simulink model "PI_Controller_sim"  (R2021a)
settings: Solver=ode23t  StartTime=0.0  StopTime=Tsim  RelTol=1e-3  EnableMultiTasking=on
values from neighbouring files (symbols this model uses):
  fo = 50    [PI_Controller.m]    (also in RL_Controller_train.m)
  Iref = 2*Pref/Vg    [PI_Controller.m]    (also in RL_Controller_train.m)
  Ka = -0.05866    [PI_Controller.m]
  Kb = 0.049031    [PI_Controller.m]
  L = 15e-3    (= 0.015)    [PI_Controller.m]    (also in RL_Controller_train.m)
  R = 1e-3    (= 0.001)    [PI_Controller.m]    (also in RL_Controller_train.m)
  Tc = 1/fpwm    (= 5e-05)    [PI_Controller.m]    (also in RL_Controller_train.m)
  Ts = 1/fs    (= 2.5e-05)    [PI_Controller.m]    (also in RL_Controller_train.m)
  Tstep = Ts/500    (= 5e-08)    [RL_Controller_train.m]
  Vdc = 400    [PI_Controller.m]    (also in RL_Controller_train.m)
  Vg = 240*sqrt(2)    [PI_Controller.m]    (also in RL_Controller_train.m)
libraries: spsIGBTDiodeLib x4, spsVoltageMeasurementLib x2, simulink x1, spsDCVoltageSourceLib x1, spsSeriesRLCBranchLib x1, spsACVoltageSourceLib x1, spsGroundLib x1, spsCurrentMeasurementLib x1, spspowerguiLib x1
settings Model: Creator=Ricardo  LastModifiedBy=ASUS-PC
settings SolverCC: AlgebraicLoopSolver=TrustRegion
settings DataIOCC: LimitDataPoints=on  SaveFormat=Array  ReturnWorkspaceOutputs=off
settings OptimizationCC: LifeSpan=inf
settings DebuggingCC: SolverPrmCheckMsg=warning  SFUnexpectedBacktrackingDiag=warning  SFNoUnconditionalDefaultTransitionDiag=warning  SFExecutionAtInitializationDiag=none  SFMachineParentedDataDiag=warning  ArithmeticOperatorsInVariantConditions=warning
settings HardwareCC: ProdBitPerPointer=32  ProdBitPerSizeT=32  ProdBitPerPtrDiffT=32  ProdLargestAtomicFloat=None  ProdIntDivRoundTo=Undefined  ProdEndianess=Unspecified  ProdWordSize=32  ProdHWDeviceType=32-bit Generic
settings ModelReferenceCC: PropagateSignalLabelsOutOfModel=off
settings SFSimCC: SimUseLocalCustomCode=off  CustomCodeUndefinedFunction=UseInterfaceOnly
settings RTWCC: RTWUseLocalCustomCode=off
settings CodeAppCC: StateflowObjectComments=on
settings GRTTargetCC: TargetLangStandard=C89/C90 (ANSI)
settings ConfigComp: CovMetricSettings=dw  CovSaveCumulativeToWorkspaceVar=on  CovSaveSingleToWorkspaceVar=on  CovExternalEMLEnable=off  CovSFcnEnable=off
settings SimscapeCC: SimscapeNormalizeSystem=off

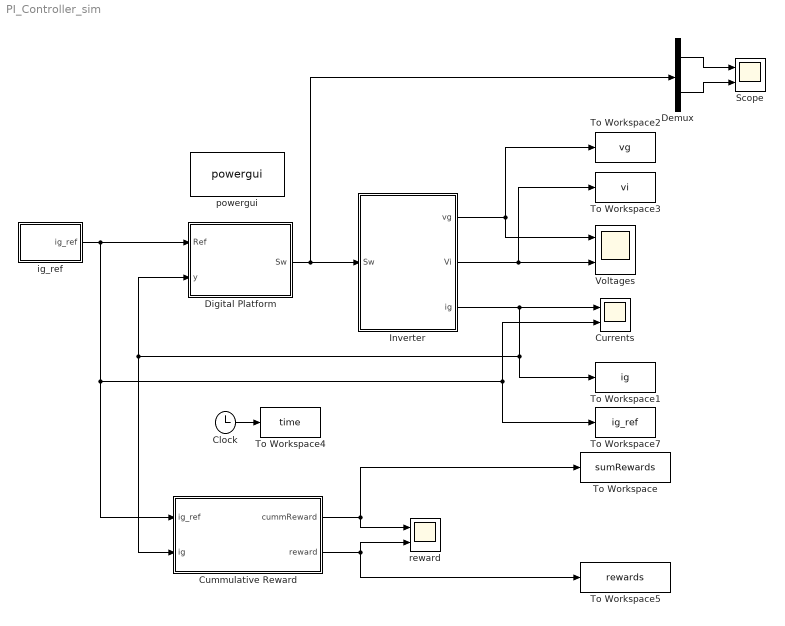
== system PI_Controller_sim ==
  Clock : Clock
  Cummulative Reward : MATLAB Function  TreatAsAtomicUnit=on  SystemSampleTime=Ts
  Currents : Scope  NumInputPorts=2
  Demux : Demux  Outputs=2
  Digital Platform : Subsystem
  Inverter : Subsystem
  Scope : Scope  NumInputPorts=2
  To Workspace : ToWorkspace  VariableName=sumRewards  SampleTime=Ts
  To Workspace1 : ToWorkspace  VariableName=ig  SampleTime=Ts
  To Workspace2 : ToWorkspace  VariableName=vg  SampleTime=Ts
  To Workspace3 : ToWorkspace  VariableName=vi  SampleTime=Ts
  To Workspace4 : ToWorkspace  VariableName=time  SampleTime=Ts
  To Workspace5 : ToWorkspace  VariableName=rewards  SampleTime=Ts
  To Workspace7 : ToWorkspace  VariableName=ig_ref  SampleTime=Ts
  Voltages : Scope  NumInputPorts=2
  ig_ref : Subsystem
  powergui : spspowerguiLib/powergui  SimulationMode=Continuous  SampleTime=Tstep  frequency=60  Iterations=50  frequencyindice=0  Pbase=100e6  ErrMax=1e-4  UnitsV=kV  UnitsW=MW  buscounter=0  FunctionMessages=off  echomessages=off  EnableUseOfTLC=off  CurrentSourceSwitches=off  DisableSnubberDevices=off  DisableRonSwitches=off  DisableVfSwitches=off  DisplayEquations=off  AutomaticDiscreteSolvers=off  SolverType=Tustin/Backward Euler (TBE)  Interpol=off  ExternalGateDelay=off  methode=off  Ts=0  x0status=blocks  SPID=off  SwTol=0  HookPort=off  NonlinearTolerance=1e-4  nMaxIteration=100  ContinueOnMaxIteration=off  RestoreLinks=warning  ResistiveCurrentMeasurement=off  Frange=[0:2:500]  Ylog=off  Xlog=on  ShowGrid=off  save=off  variable=ZData  structure=Currents  ZoomFFT=off  StartTime=0.0  cycles=2  DisplayStyle=4  fundamental=50  FreqAxis=off  MaxFrequency=2500  frequencyindicesteady=1  RmsSteady=1  display=off
  reward : Scope  NumInputPorts=2
  wires:
  Clock/1 -> To Workspace4/1
  Inverter/1(vg) -> Voltages/1, To Workspace2/1
  Inverter/2(Vi) -> Voltages/2, To Workspace3/1
  Inverter/3(ig) -> Cummulative Reward/2(ig), Digital Platform/2(y), To Workspace1/1, Currents/1
  ig_ref/1(ig_ref) -> Cummulative Reward/1(ig_ref), Currents/2, To Workspace7/1, Digital Platform/1(Ref)
  Digital Platform/1(Sw) -> Demux/1, Inverter/1(Sw)
  Demux/1 -> Scope/1
  Demux/2 -> Scope/2
  Cummulative Reward/2(reward) -> reward/2, To Workspace5/1
  Cummulative Reward/1(cummReward) -> reward/1, To Workspace/1

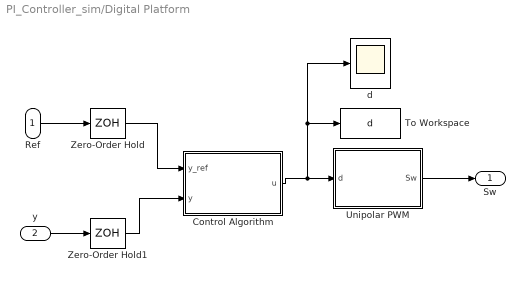
== system PI_Controller_sim/Digital Platform ==
  Ref : Inport
  y : Inport  Port=2
  Control Algorithm : MATLAB Function  TreatAsAtomicUnit=on
  To Workspace : ToWorkspace  VariableName=d  SampleTime=Ts
  Unipolar PWM : Subsystem
  Zero-Order Hold : ZeroOrderHold  SampleTime=Ts
  Zero-Order Hold1 : ZeroOrderHold  SampleTime=Ts
  d : Scope
  Sw : Outport  VectorParamsAs1DForOutWhenUnconnected=off
  wires:
  Zero-Order Hold1/1 -> Control Algorithm/2(y)
  y/1 -> Zero-Order Hold1/1
  Zero-Order Hold/1 -> Control Algorithm/1(y_ref)
  Ref/1 -> Zero-Order Hold/1
  Unipolar PWM/1(Sw) -> Sw/1
  Control Algorithm/1(u) -> d/1, To Workspace/1, Unipolar PWM/1(d)

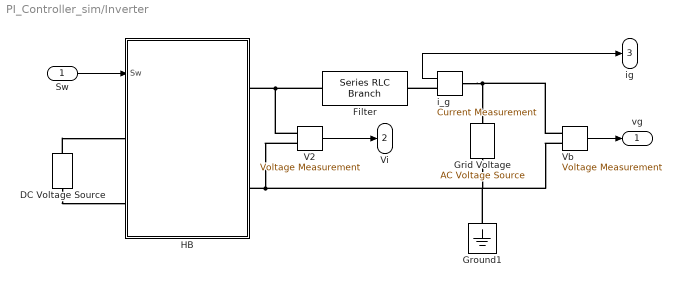
== system PI_Controller_sim/Inverter ==
  Sw : Inport
  DC Voltage Source : spsDCVoltageSourceLib/DC Voltage Source  Amplitude=Vdc  Measurements=None
  Filter : spsSeriesRLCBranchLib/Series RLC Branch  LConnTagsString=__new0  RConnTagsString=__new0  BranchType=RL  Resistance=R  Inductance=L  SetiL0=on  InitialCurrent=0  Capacitance=1e-6  Setx0=off  InitialVoltage=0  Measurements=Branch current
  Grid Voltage : spsACVoltageSourceLib/AC Voltage Source  Amplitude=Vg  Phase=0  Frequency=fo  SampleTime=0  Measurements=None  BusType=swing  Pref=10e3  Qref=0  Qmin=-inf  Qmax=+inf
  Ground1 : spsGroundLib/Ground  LConnTagsString=a
  HB : Subsystem
  V2 : spsVoltageMeasurementLib/Voltage Measurement  Tag=PoWeRsYsTeMmEaSuReMeNt  PhasorSimulation=off  OutputType=Magnitude  PSBequivalent=0
  Vb : spsVoltageMeasurementLib/Voltage Measurement  Tag=PoWeRsYsTeMmEaSuReMeNt  PhasorSimulation=off  OutputType=Magnitude  PSBequivalent=0
  i_g : spsCurrentMeasurementLib/Current Measurement  PhasorSimulation=off  OutputType=Complex  PSBequivalent=0
  vg : Outport  VectorParamsAs1DForOutWhenUnconnected=off
  Vi : Outport  Port=2  VectorParamsAs1DForOutWhenUnconnected=off
  ig : Outport  Port=3  VectorParamsAs1DForOutWhenUnconnected=off
  wires:
  Vb/1 -> vg/1
  Sw/1 -> HB/1(Sw)
  V2/1 -> Vi/1
  i_g/1 -> ig/1
  connections:
  DC Voltage Source/RConn1 -- HB/LConn1
  Vb/LConn1 -- Grid Voltage/RConn1 -- i_g/LConn1
  V2/LConn1 -- Filter/LConn1 -- HB/RConn1
  V2/LConn2 -- Grid Voltage/LConn1 -- Vb/LConn2 -- Ground1/LConn1 -- HB/RConn2
  DC Voltage Source/LConn1 -- HB/LConn2
  i_g/RConn1 -- Filter/RConn1

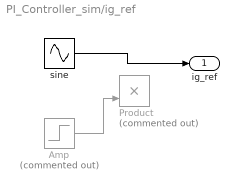
== system PI_Controller_sim/ig_ref ==
  Amp : Step  Commented=on  Time=0.055  Before=Iref  After=-Iref  SampleTime=0
  Product : Product  Commented=on
  sine : Sin  Amplitude=Iref  Frequency=2*pi*fo  SampleTime=0
  ig_ref : Outport  VectorParamsAs1DForOutWhenUnconnected=off
  wires:
  Amp/1 -> Product/2
  sine/1 -> ig_ref/1

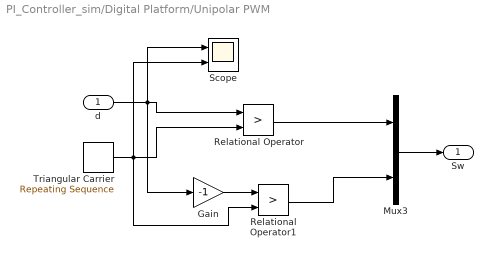
== system PI_Controller_sim/Digital Platform/Unipolar PWM ==
  d : Inport
  Gain : Gain  Gain=-1
  Mux3 : Mux  Inputs=2
  Relational Operator : RelationalOperator  Operator=>  OutDataTypeStr=boolean  RndMeth=Simplest  InputSameDT=on
  Relational Operator1 : RelationalOperator  Operator=>  OutDataTypeStr=boolean  RndMeth=Simplest  InputSameDT=on
  Scope : Scope  NumInputPorts=2
  Triangular Carrier : simulink/Sources/Repeating Sequence  rep_seq_t=[0 Tc 2*Tc]  rep_seq_y=[0 1 0]
  Sw : Outport  VectorParamsAs1DForOutWhenUnconnected=off
  wires:
  Mux3/1 -> Sw/1
  d/1 -> Scope/1, Gain/1, Relational Operator/1
  Triangular Carrier/1 -> Scope/2, Relational Operator1/2, Relational Operator/2
  Gain/1 -> Relational Operator1/1
  Relational Operator/1 -> Mux3/1
  Relational Operator1/1 -> Mux3/2

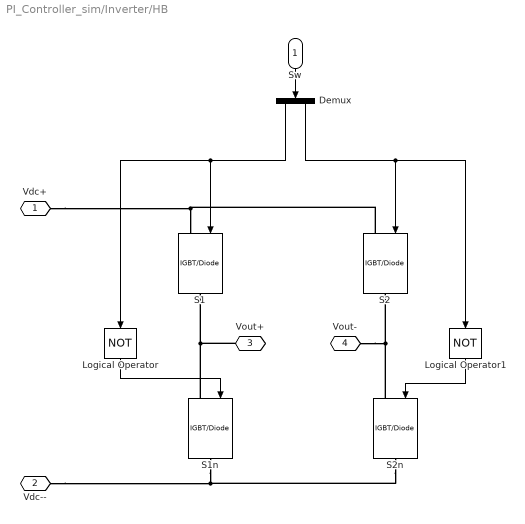
== system PI_Controller_sim/Inverter/HB ==
  Sw : Inport
  Demux : Demux  Outputs=2
  Logical Operator : Logic  Operator=NOT  AllPortsSameDT=off  OutDataTypeStr=boolean
  Logical Operator1 : Logic  Operator=NOT  AllPortsSameDT=off  OutDataTypeStr=boolean
  S1 : spsIGBTDiodeLib/IGBT//Diode  Ron=1e-3  Rs=1e5  Cs=inf  Measurements=off
  S1n : spsIGBTDiodeLib/IGBT//Diode  Ron=1e-3  Rs=1e5  Cs=inf  Measurements=off
  S2 : spsIGBTDiodeLib/IGBT//Diode  Ron=1e-3  Rs=1e5  Cs=inf  Measurements=off
  S2n : spsIGBTDiodeLib/IGBT//Diode  Ron=1e-3  Rs=1e5  Cs=inf  Measurements=off
  Vdc+ : PMIOPort  Side=Left
  Vdc-- : PMIOPort  Port=2  Side=Left
  Vout+ : PMIOPort  Port=3  Side=Right
  Vout- : PMIOPort  Port=4  Side=Right
  wires:
  Logical Operator/1 -> S1n/1
  Sw/1 -> Demux/1
  Demux/1 -> Logical Operator/1, S1/1
  Logical Operator1/1 -> S2n/1
  Demux/2 -> Logical Operator1/1, S2/1
  connections:
  S1n/RConn1 -- Vdc--/RConn1 -- S2n/RConn1
  S1n/LConn1 -- Vout+/RConn1 -- S1/RConn1
  S2n/LConn1 -- Vout-/RConn1 -- S2/RConn1
  S2/LConn1 -- Vdc+/RConn1 -- S1/LConn1

== matlab function PI_Controller_sim/Cummulative Reward ==
  data: ig_ref input; cummReward output; ig input; reward output
function [cummReward, reward]= calcReward(ig_ref, ig)

    persistent sumReward;
    if isempty(sumReward)
        sumReward = 0;
    end
    
    % reward on this time step
    reward = abs(ig_ref-ig)*-0.1;
    
    % cummulative reward
    sumReward = sumReward+reward;
    
    % output to view on scope
    cummReward = sumReward;
end

== matlab function PI_Controller_sim/Digital Platform/Control Algorithm ==
  data: y_ref input; y input; u output; Ka parameter; Kb parameter
function u = DCtrl(y_ref,y,Ka, Kb)  
% You can add more parameters to be read from the workspace like Ka, Kb
% For extra parameters, just be sure to define them as parameters in 
% "Edit Data", next to "Build Model.
%
% Check the screenshot in "Adding_Parameters_to_Matlab_Function.PDF"
%% Variables

%%Memories 
%e(k-1)
persistent e_k_1   
if isempty(e_k_1)
    e_k_1=0;        %Initial value for e(k-1)=0
end
%u(k-1)
persistent u_k_1   
if isempty(u_k_1)
    u_k_1=0;        %Initial value for u(k-1)=0
end

%% Digital controller
%Implement here your controller
e_k=y_ref-y;

%u(k)=Ka*e(k)+Kb*e(k-1)+u(k-1)
u_k=Ka*e_k+Kb*e_k_1+u_k_1;    

%% Anti-windup: duty-cycle between -1 to 1
if (u_k>1)
    u_k=1;
elseif (u_k<-1)
    u_k=-1;
end

%% Variable updates
e_k_1=e_k;
u_k_1=u_k;

%% Input to be applied to the plant
u=u_k;
